simulink model "StateSpaceResults"  (R2023a)
settings: Solver=VariableStepAuto  StartTime=0.0  StopTime=100  RelTol=1e-3
undefined symbols (not defined in the file): X_den, X_num, Y_den, Y_num
settings Model: Creator=minim  LastModifiedBy=minim

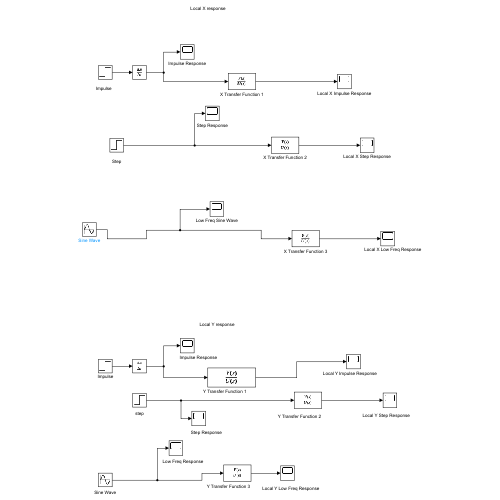
[thumbnail: Simulink's stored preview of the top-level diagram]
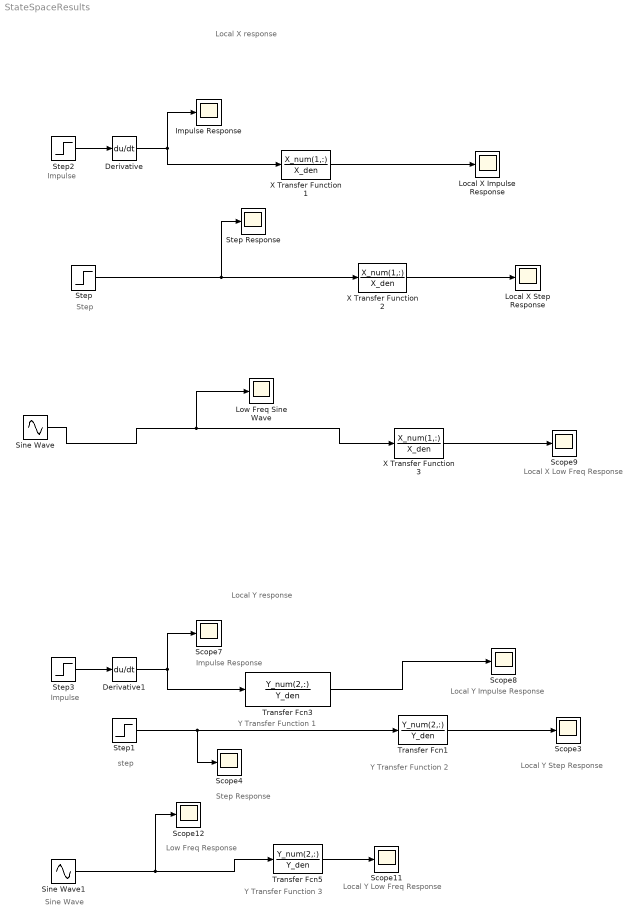
== system StateSpaceResults ==
  note: Y Transfer Function 3
  note: Y Transfer Function 2
  note: Y Transfer Function 1
  note: Sine Wave
  note: Local Y Low Freq Response
  note: Local Y Step Response
  note: Local Y Impulse Response
  note: Local X Low Freq Response
  note: Impulse
  note: Local Y response
  note: Step
  note: step
  note: Impulse Response
  note: Local X response
  note: Impulse
  note: Step Response
  note: Low Freq Response
  Derivative : Derivative  CoefficientInTFapproximation=0
  Derivative1 : Derivative  CoefficientInTFapproximation=0
  Impulse Response : Scope
  Local X Impulse Response : Scope
  Local X Step Response : Scope
  Low Freq Sine Wave : Scope
  Scope{3..4,7..9,11..12} (7 alike) : Scope
  Sine Wave : Sin  Frequency=0.01  SampleTime=0  VectorParams1D=off
  Sine Wave1 : Sin  SampleTime=0  VectorParams1D=off
  Step : Step  After=0.1  SampleTime=0
  Step Response : Scope
  Step1 : Step  After=0.1  SampleTime=0
  Step2 : Step  SampleTime=0
  Step3 : Step  SampleTime=0
  Transfer Fcn1 : TransferFcn  Numerator=Y_num(2,:)  Denominator=Y_den
  Transfer Fcn3 : TransferFcn  Numerator=Y_num(2,:)  Denominator=Y_den
  Transfer Fcn5 : TransferFcn  Numerator=Y_num(2,:)  Denominator=Y_den
  X Transfer Function 1 : TransferFcn  Numerator=X_num(1,:)  Denominator=X_den
  X Transfer Function 2 : TransferFcn  Numerator=X_num(1,:)  Denominator=X_den
  X Transfer Function 3 : TransferFcn  Numerator=X_num(1,:)  Denominator=X_den
  wires:
  Step2/1 -> Derivative/1
  Derivative/1 -> Impulse Response/1, X Transfer Function 1/1
  X Transfer Function 1/1 -> Local X Impulse Response/1
  Step/1 -> X Transfer Function 2/1, Step Response/1
  Step3/1 -> Derivative1/1
  X Transfer Function 2/1 -> Local X Step Response/1
  Transfer Fcn1/1 -> Scope3/1
  Step1/1 -> Transfer Fcn1/1, Scope4/1
  Derivative1/1 -> Scope7/1, Transfer Fcn3/1
  Transfer Fcn3/1 -> Scope8/1
  Sine Wave/1 -> X Transfer Function 3/1, Low Freq Sine Wave/1
  X Transfer Function 3/1 -> Scope9/1
  Transfer Fcn5/1 -> Scope11/1
  Sine Wave1/1 -> Transfer Fcn5/1, Scope12/1
